simulink library "Trap_lib"  (R2019a)
settings: Solver=VariableStepAuto  StartTime=0.0  StopTime=10.0  RelTol=1e-3
values from neighbouring files (symbols this model uses):
  dt = 1*10^-4    (= 0.0001)    [initMonteCarlo.m]    (also in initRealModel.m = 0.001; initTrapModel.m = 1e-05)
  RTrap = 0.0011    [initTrapModel.m]
settings Model: Creator=martin  LastModifiedBy=martin

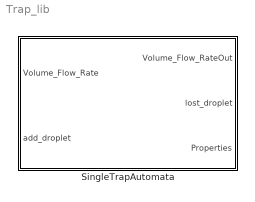
== system Trap_lib ==
  SingleTrapAutomata : Subsystem  mask{width=0, length=0, height=0, Rtrap=RTrap, dt=dt}
      mask prompts: width "Pipe Width"; length "Pipe Length"; height "Pipe Height"; Rtrap "resistance of trap if filled"; dt "time step"
      mask TypeOptions Rtrap: Custom_Integrator/Rtrap
      mask TypeOptions dt: Custom_Integrator/dt

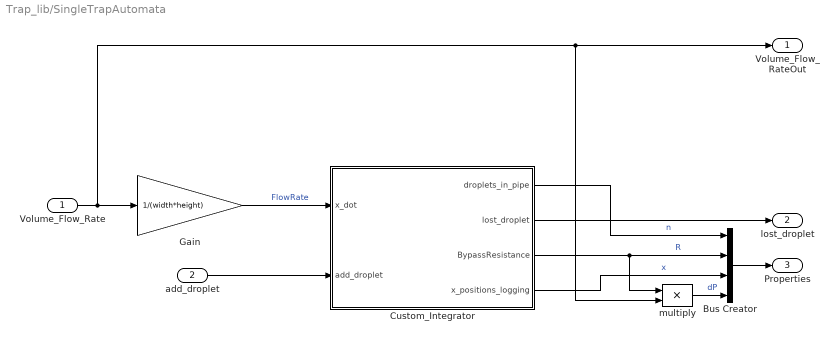
== system Trap_lib/SingleTrapAutomata ==
  Volume_Flow_Rate : Inport
  add_droplet : Inport  Port=2
  Bus Creator : BusCreator  Inputs=4
  Custom_Integrator : MATLAB Function  TreatAsAtomicUnit=on  mask{dt=dt, upper_Limit=length, Rtrap=Rtrap, Rc=3*(12*(1-(192*height)/(width*pi^5)*tanh((pi*width)/(2*height)))^-1)*length/(width*height^3)*0.001, Rd=(12*(1-(192*height)/(width*pi^5)*tanh((pi*width)/(2*height)))^-1)*length/(width*height^3)*0.001}
      mask prompts: dt "time step"; upper_Limit "bypass length"; Rtrap "resistance of trap if filled"; Rc "reistance of pipe without droplets"; Rd "resistance per droplet"
  Gain : Gain  Gain=1/(width*height)
  multiply : Product  Inputs=**
  Volume_Flow_RateOut : Outport
  lost_droplet : Outport  Port=2
  Properties : Outport  Port=3
  wires:
  Gain/1 -> Custom_Integrator/1(x_dot)  "FlowRate"
  add_droplet/1 -> Custom_Integrator/2(add_droplet)
  Custom_Integrator/2(lost_droplet) -> lost_droplet/1
  Custom_Integrator/1(droplets_in_pipe) -> Bus Creator/1  "n"
  Custom_Integrator/4(x_positions_logging) -> Bus Creator/3  "x"
  Custom_Integrator/3(BypassResistance) -> multiply/1, Bus Creator/2  "R"
  Volume_Flow_Rate/1 -> multiply/2, Volume_Flow_RateOut/1, Gain/1
  Bus Creator/1 -> Properties/1
  multiply/1 -> Bus Creator/4  "dP"

== matlab function Trap_lib/SingleTrapAutomata/Custom_Integrator ==
  data: x_dot input; dt parameter; add_droplet input; upper_Limit parameter; droplets_in_pipe output size=[1,2]; lost_droplet output; BypassResistance output; x_positions_logging output size=10; Rc parameter; Rd parameter; Rtrap parameter
function [droplets_in_pipe, lost_droplet, BypassResistance, x_positions_logging] = fcn(x_dot, dt, add_droplet, upper_Limit, Rc, Rd, Rtrap)

%% declare persistent memory/internal state
persistent x_state
persistent trap_state
persistent number_droplet
%% initalize internal state/memory 
if (isempty(x_state))
    x_state = [];
end
if (isempty(number_droplet))
    number_droplet = 0;
end
if (isempty(trap_state))
    trap_state = 0;
end

%% first check if we added a new droplet to the trap
if(add_droplet > 0)
    if (trap_state > 0)    
        number_droplet = number_droplet+1;
        x_state = [x_state,0];
    else
        trap_state = trap_state + 1;
    end
end

%% calc resistances
BypassResistance = Rc + number_droplet*Rd;
TrapResistance = Rtrap * trap_state;
lost_droplet_trap = 0;
if (BypassResistance > TrapResistance && add_droplet > 0)
    lost_droplet_trap = 1;
    trap_state = 0;
end

%% now propegate droplet position in bypass pipe
% use first order integration
if (number_droplet>0)
    x_state = x_state + repmat(x_dot, 1, numel(x_state))*dt;
end

%% check if any droplets left the pipe
index = x_state > upper_Limit;
x_state = x_state(~index);
lost_droplet_bypass = sum(index);

switch lost_droplet_bypass
    case 0
        droplets_in_pipe = [trap_state,number_droplet];
    case 1
        number_droplet = number_droplet - lost_droplet_bypass;
        droplets_in_pipe = [trap_state,number_droplet];
    otherwise
        error('out side of valid dynamics, reduce step size to prevent two droplets leaving at the same time')
end

lost_droplet = lost_droplet_bypass + lost_droplet_trap;
if (lost_droplet > 1)
    error('out side of valid dynamics, reduce step size to prevent two droplets leaving at the same time')
end

%% Add position output for debug
x_positions_logging = zeros(10,1);

index_log = min([10,number_droplet]);

x_positions_logging(1:index_log) = x_state(1:index_log);
